simulink model "Simulate"  (R2024b)
settings: Solver=VariableStepAuto  StartTime=0.0  StopTime=Tf  FixedStep=Ti  MaxStep=Ti  RelTol=1e-6
undefined symbols (not defined in the file): CCMPC, CEMPC, DiscIntNeverNeededParam, dspblkCoreblockFVToolHelper, FOC, gcbh, IM, KF, LPF, M2C, plecs, PLL, RFT, TEB, Ti, Ts
libraries: slpidlib x4, spsdq0toAlphaBetaZeroLib x3, dspstat3 x2, spsAlphaBetaZerotoabcLib x2, embmathops x1, spsabctodq0Lib x1, spsAlphaBetaZerotodq0Lib x1, spsabctoAlphaBetaZeroLib x1
(part 2 of 2)

== matlab function Simulate/Energy balance1 ==
  data: Ec input; Vc input; VB input; IB input; ie_ref output; vo_ref output; flag output; J output; Nac output; Tex output; M2C parameter; CEMPC parameter
function [ie_ref, vo_ref, flag, J, Nac, Tex] = EMPC(Ec, Vc, VB, IB, M2C, CEMPC)
%#codegen

persistent Ts m n Np K MI NN NN1 NN2 ONE Nl is_max Vc_m_ref2 Ec_m_ref2 Hu_z1 Aineq_z1 Hu_z2 Aineq_z2 Hu_o Aineq_o lambda_z lambda_o iA_z1 iA_z2 iA_o options_z options_o
if isempty(Ts)
    Ts        = CEMPC.Ts;
    m         = M2C.m;
    n         = M2C.n;
    Np        = CEMPC.Np;
    K         = CEMPC.K;
    MI        = CEMPC.MI;
    NN        = CEMPC.NN;
    NN1       = CEMPC.NN1;
    NN2       = CEMPC.NN2;
    ONE       = CEMPC.ONE;
    Nl        = CEMPC.Nl;
    is_max    = M2C.is_max;
    Vc_m_ref2 = M2C.Vc_m_ref^2;
    Ec_m_ref2 = M2C.Ec_m_ref^2;
    Hu_z1     = CEMPC.Hu_z1;
    Aineq_z1  = CEMPC.Aineq_z1;
    Hu_z2     = CEMPC.Hu_z2;
    Aineq_z2  = CEMPC.Aineq_z2;
    Hu_o      = CEMPC.Hu_o;
    Aineq_o   = CEMPC.Aineq_o;
    lambda_z  = CEMPC.lambda_z;
    lambda_o  = CEMPC.lambda_o;
    iA_z1     = false(size(zeros(2 * m * Np, 1)));
    iA_z2     = false(size(zeros(2 * m * Np, 1)));
    iA_o      = false(size(zeros(2 * Np, 1)));
    options_z                     = mpcActiveSetOptions;
    options_z.MaxIterations       = 20;
    options_z.ConstraintTolerance = 1e-4;
    options_o                     = mpcActiveSetOptions;
    options_o.MaxIterations       = 10;
    options_o.ConstraintTolerance = 1e-4;
end

tic

% Preallocation
vo_ref_temp = zeros(Np, 1);
ie_ref_temp = zeros(n*Np, 1);
ie1_ref_temp = zeros(Np, 1);
ie2_ref_temp = zeros(Np, 1);
iz1_ref_temp = zeros(m*Np, 1);
iz2_ref_temp = zeros(m*Np, 1);
flag_z1 = int32(0);
flag_z2 = int32(0);
flag_o = int32(0);
vs_temp = zeros(m*Np, 1);
is_temp = zeros(m*Np, 1);

for l = 1:Nl
    %%%% LICCs subproblems J_z1 = Jx_z1 + Ju_z1, J_z2 = Jx_z2 + Ju_z2

    % Initialization
    vs_temp(:) = VB(:) + ONE * vo_ref_temp; % Cluster voltages

    %%% 1st LICC
    % Initialization
    iz2_ref_temp = NN2 * ie2_ref_temp; % 2nd circulating current

    % Linear model matrices
    E = Ts * K * diag(vs_temp); % Disturbances matrix
    B = E * NN1;                % Input matrix
    P = IB(:) + iz2_ref_temp;   % Disturbances

    % State reference tracking Jx_z1, quadratic and linear terms
    Hx_z1 = 2 * B' * MI * B / Ec_m_ref2;
    fx_z1 = 2 * B' * MI * (repmat(Ec, Np, 1) + E * P) / Ec_m_ref2;

    % Control action penalization Ju_z1, linear term
    fu_z1 = 2 * NN1' * P / is_max^2;

    % Total cost function J_z
    H_z1 = Hx_z1 + lambda_z * Hu_z1;
    f_z1 = fx_z1 + lambda_z * fu_z1;
    H_z1 = (H_z1 + H_z1') / 2;

    % Constraints
    ub      =  is_max - P;
    lb      = -is_max - P;
    bineq_z1 = [ub; -lb];

    % Solve
    [ie1_ref_temp, flag_z1, iA_z1] = mpcActiveSetSolver(H_z1, f_z1, Aineq_z1, bineq_z1, zeros(0, Np), zeros(0, 1), iA_z1, options_z);

    %%% 2nd LICC
    % Initialization
    iz1_ref_temp = NN1 * ie1_ref_temp; % 1nd circulating current

    % Linear model matrices
    E = Ts * K * diag(vs_temp); % Disturbances matrix
    B = E * NN2;                % Input matrix
    P = IB(:) + iz1_ref_temp;   % Disturbances

    % State reference tracking Jx_z2, quadratic and linear terms
    Hx_z2 = 2 * B' * MI * B / Ec_m_ref2;
    fx_z2 = 2 * B' * MI * (repmat(Ec, Np, 1) + E * P) / Ec_m_ref2;

    % Control action penalization Ju_z2, linear term
    fu_z2 = 2 * NN2' * P / is_max^2;

    % Total cost function J_z
    H_z2 = Hx_z2 + lambda_z * Hu_z2;
    f_z2 = fx_z2 + lambda_z * fu_z2;
    H_z2 = (H_z2 + H_z2') / 2;

    % Constraints
    ub       =  is_max - P;
    lb       = -is_max - P;
    bineq_z2 = [ub; -lb];

    % Solve
    [ie2_ref_temp, flag_z2, iA_z2] = mpcActiveSetSolver(H_z2, f_z2, Aineq_z2, bineq_z2, zeros(0, Np), zeros(0, 1), iA_z2, options_z);

    %%%% CMV subproblem Jo = Jx_o + Ju_o

    % Initialization
    iz1_ref_temp = NN1 * ie1_ref_temp;
    iz2_ref_temp = NN2 * ie2_ref_temp;
    iz_ref_temp = iz1_ref_temp + iz2_ref_temp;
    is_temp = IB(:) + iz_ref_temp;

    % Linear model matrices
    E = Ts * K * diag(is_temp); % Distrubances matrix
    B = E * ONE;                % Input matrix
    P = VB(:);                  % Distrubances

    % State reference tracking Jx_o, quadratic and linear terms 
    Hx_o = 2 * B' * MI * B / Ec_m_ref2;
    fx_o = 2 * B' * MI * (repmat(Ec, Np, 1) + E * P) / Ec_m_ref2;

    % Control action penalization Jo_u
    fu_o = zeros(Np, 1) / Vc_m_ref2;

    % Total cost function J_o
    H_o = Hx_o + lambda_o * Hu_o;
    f_o = fx_o + lambda_o * fu_o;
    H_o = (H_o + H_o') / 2;

    % Constraints
    ub = min([Vc(1:3); 0; 0; 0] - VB, [], 1)';
    lb = max([0; 0; 0; -Vc(4:6)] - VB, [], 1)';
    bineq_o = [ub; -lb];

    % Solve
    [vo_ref_temp, flag_o, iA_o] = mpcActiveSetSolver(H_o, f_o, Aineq_o, bineq_o, zeros(0, Np), zeros(0, 1), iA_o, options_o);
end

% ie_ref = ie_ref_temp(1:n);
ie_ref = ie_ref_temp(1:2);
vo_ref = vo_ref_temp(1);

vs_temp = VB(:) + ONE * vo_ref_temp;
Ec_pred = Ec + Ts * reshape(vs_temp .* is_temp, m, Np);
Ec_pred = Ec_pred(:);
J_E = sum((Ec_pred - mean(Ec_pred)).^2) / Ec_m_ref2;
J_i = sum(is_temp.^2) / is_max^2;
J_v = sum(vo_ref_temp.^2) / Vc_m_ref2;
J_T = J_E + lambda_z * J_i + lambda_o * J_v;

flag = [flag_z1, flag_z2, flag_o];
J = [J_E, J_i, J_v, J_T];
Nac = [sum(iA_z1), sum(iA_z2), sum(iA_o)];

Tex = toc;
end

% Hx = 2 * B' * B / M2C.Ec_m_ref^2;
% fx = 2 * B' * (repmat(x-mean(x), CEMPC.Np, 1) + E * P) / M2C.Ec_m_ref^2;

== matlab function Simulate/M2C+IM Average Model ==
  data: vs input; vB input; Fr_ab input; wm input; iu output; M2C parameter; CCMPC parameter; im output; ie output; Vc output; RFT parameter
function [iu, im, ie, Vc] = DM2C(vs, vB, Fr_ab, wm, M2C, CCMPC, RFT)

% DM2C: Decoupled M2C

persistent Ec m nx x Ad Bd integrated Tab2abc pinvA N Vdc Ts C
if isempty(Ec)
    m = M2C.m;
    Ec = M2C.Ec_m_ref * ones(m, 1);
    nx = CCMPC.nx;
    x = zeros(nx, 1);
    Ad = CCMPC.Ad;
    Bd = CCMPC.Bd;
    integrated = CCMPC.integrated;
    Tab2abc = RFT.ab2abc;
    pinvA = M2C.pinvA;
    N = M2C.N;
    Vdc = M2C.Vdc;
    Ts = CCMPC.Ts;
    C = M2C.C;
end

Es = CCMPC.Es;
Es(2, 3) = Es(2, 3)*wm;
Es(3, 2) = Es(3, 2)*wm;
Ed = integrated*Es;

p = [Vdc;
     Fr_ab;
     vB];

x = Ad * x + Bd * vs + Ed * p;

iu = x(1);
im = Tab2abc * x(2:3);
ie = x(2:3);

ixy = [iu;
      -iu;
      -im];
iB = pinvA * ixy;
iz = N * ie;
is = iB + iz;

Ec = Ec + Ts * vs .* is;

Vc = zeros(6, 1);
Vc(:) = sqrt(2 / C * Ec);

== matlab function Simulate/Energy balance ==
  data: Ec input; Vc input; VB input; IB input; ie_ref output; vo_ref output; flag output; J output; Nac output; Tex output; M2C parameter; CEMPC parameter
function [ie_ref, vo_ref, flag, J, Nac, Tex] = EMPC(Ec, Vc, VB, IB, M2C, CEMPC)
%#codegen

persistent Ts m n Np K MI NN ONE Nl is_max Vc_m_ref2 Ec_m_ref2 Hu_z Aineq_z lambda_z Hu_o Aineq_o lambda_o iA_z iA_o options_z options_o
if isempty(iA_z)
    Ts        = CEMPC.Ts;
    m         = M2C.m;
    n         = M2C.n;
    Np        = CEMPC.Np;
    K         = CEMPC.K;
    MI        = CEMPC.MI;
    NN        = CEMPC.NN;
    ONE       = CEMPC.ONE;
    Nl        = CEMPC.Nl;
    is_max    = M2C.is_max;
    Vc_m_ref2 = M2C.Vc_m_ref^2;
    Ec_m_ref2 = M2C.Ec_m_ref^2;
    Hu_z      = CEMPC.Hu_z;
    Aineq_z   = CEMPC.Aineq_z;
    lambda_z  = CEMPC.lambda_z;
    Hu_o      = CEMPC.Hu_o;
    Aineq_o   = CEMPC.Aineq_o;
    lambda_o  = CEMPC.lambda_o;
    iA_z      = false(size(zeros(2 * m * Np, 1)));
    iA_o      = false(size(zeros(2 * Np, 1)));
    options_z                     = mpcActiveSetOptions;
    options_z.MaxIterations       = 20;
    options_z.ConstraintTolerance = 1e-4;
    options_o                     = mpcActiveSetOptions;
    options_o.MaxIterations       = 10;
    options_o.ConstraintTolerance = 1e-4;
end

tic

% Preallocation
vo_ref_temp = zeros(Np, 1);
ie_ref_temp = zeros(n*Np, 1);
flag_z = int32(0);
flag_o = int32(0);
vs_temp = zeros(m*Np, 1);
is_temp = zeros(m*Np, 1);

for l = 1:Nl
    %%% LICCs subproblem Jz = Jz_x + Jz_u

    % Initialization
    % vs_temp(:) = VB(:) + ONE * vo_ref_temp;
    vs_temp = VB + vo_ref_temp';
    vs_temp = vs_temp(:);

    % Linear model matrices
    E = Ts * K * diag(vs_temp); % Disturbances matrix
    B = E * NN;                 % Input matrix
    P = IB(:);                  % Disturbances

    % State reference tracking Jx_z, quadratic and linear terms 
    Hx_z = 2 * B' * MI * B / Ec_m_ref2;
    fx_z = 2 * B' * MI * (repmat(Ec, Np, 1) + E * P) / Ec_m_ref2;

    % Control action penalization Ju_z, linear term
    fu_z = 2 * NN' * IB(:) / is_max^2;

    % Total cost function J_z
    H_z = Hx_z + lambda_z * Hu_z;
    f_z = fx_z + lambda_z * fu_z;
    H_z = (H_z + H_z') / 2;

    % Constraints
    ub      =  is_max - IB(:);
    lb      = -is_max - IB(:);
    bineq_z = [ub; -lb];

    % Solve
    [ie_ref_temp, flag_z, iA_z] = mpcActiveSetSolver(H_z, f_z, Aineq_z, bineq_z, zeros(0, n*Np), zeros(0, 1), iA_z, options_z);

    %%% CMV subproblem Jo = Jo_x + Jo_u

    % Initialization
    is_temp = IB(:) + NN * ie_ref_temp;

    % Linear model matrices
    E = Ts * K * diag(is_temp); % Distrubances matrix
    B = E * ONE;                % Input matrix
    P = VB(:);                  % Distrubances

    % State reference tracking Jx_o, quadratic and linear terms 
    Hx_o = 2 * B' * MI * B / Ec_m_ref2;
    fx_o = 2 * B' * MI * (repmat(Ec, Np, 1) + E * P) / Ec_m_ref2;

    % Control action penalization Jo_u
    fu_o = zeros(Np, 1) / Vc_m_ref2;

    % Total cost function J_o
    H_o = Hx_o + lambda_o * Hu_o;
    f_o = fx_o + lambda_o * fu_o;
    H_o = (H_o + H_o') / 2;

    % Constraints
    ub = min([Vc(1:3); 0; 0; 0] - VB, [], 1)';
    lb = max([0; 0; 0; -Vc(4:6)] - VB, [], 1)';
    bineq_o = [ub; -lb];

    % Solve
    [vo_ref_temp, flag_o, iA_o] = mpcActiveSetSolver(H_o, f_o, Aineq_o, bineq_o, zeros(0, Np), zeros(0, 1), iA_o, options_o);
end

% ie_ref = ie_ref_temp(1:n);
ie_ref = ie_ref_temp(1:2);
vo_ref = vo_ref_temp(1);

if and(0 < flag_z, 0 < flag_o)
    flag_T = 1;
else
    flag_T = -3;
end

vs_temp = VB(:) + ONE * vo_ref_temp;
Ec_pred = Ec + Ts * reshape(vs_temp .* is_temp, m, Np);
Ec_pred = Ec_pred(:);
J_E = sum((Ec_pred - mean(Ec_pred)).^2) / Ec_m_ref2;
J_i = sum(is_temp.^2) / is_max^2;
J_v = sum(vo_ref_temp.^2) / Vc_m_ref2;
J_T = J_E + lambda_z * J_i + lambda_o * J_v;

flag = [flag_z, flag_o, flag_T];
J = [J_E, J_i, J_v, J_T];
Nac = [sum(iA_z), sum(iA_o)];

Tex = toc;
end

== matlab function Simulate/Subsystem/MATLAB Function ==
  data: Vc input; vo_max output; vB input; vo_min output
function [vo_max, vo_min] = vo_lim(Vc, vB)

vo_max = min([Vc(1:3); zeros(3, 1)] - vB);
vo_min = max([zeros(3, 1); -Vc(4:6)] - vB);

== matlab function Simulate/Current control Converter only ==
  data: is_ref input; vo_ref input; vs_ref input; is input; vs output; Vc input; vB input; flag output; J output; Nac output; Tex output; M2C parameter; CCMPC parameter
function [vs, flag, J, Nac, Tex] = CMPC(is_ref, vo_ref, vs_ref, is, Vc, vB, M2C, CCMPC)
%#codegen

% CMPC: Cluster Current Model Predictive Control

% vs:   control action
% flag: solver verbose
% J:    cost function
% Nac:  # of active constraints
% Tex:  Execution time

% Initialization

persistent Ad Bd is_max Vc_m_ref lambda m Hx Hu H Aineq iA options
if isempty(Ad)
    Ad       = CCMPC.Ad;                  % Discrete state matrix
    Bd       = CCMPC.Bd;                  % Discrete input matrix
    is_max   = M2C.is_max;                % Max. cluster current
    Vc_m_ref = M2C.Vc_m_ref;              % Max. cluster capacitor voltage
    lambda   = CCMPC.lambda;              % Control effort weighting factor
    m        = M2C.m;                     % # of converter clusters
    Hx       = CCMPC.Hx;                  % Reference tracking hessian
    Hu       = CCMPC.Hu;                  % Control effort hessian
    H        = CCMPC.H;                   % Total hessian
    Aineq    = CCMPC.Aineq;               % Control actions constraints matrix
    iA       = false(size(Aineq, 1), 1);  % Active constraints
    options  = mpcActiveSetOptions;       % mpcActiveSetSolver options
    options.MaxIterations       = 100;
    options.ConstraintTolerance = 1.0e-5;
end

tic

% Reference tracking linear term, normalized
fx = 2 * Bd' * (-is_ref + Ad * is - Bd * vB) / is_max^2;

% Control effort linear term, normalized
fu = -2 * vs_ref / Vc_m_ref^2;

% Total weighted linear term
f = fx + lambda * fu;

% Control action constraints
ub    = [Vc(1:3); 0; 0; 0] + vo_ref;
lb    = [0; 0; 0; -Vc(4:6)] + vo_ref;
bineq = [ub; -lb];

% Solve
[vsp, flag, iA, ~] = mpcActiveSetSolver(H, f, Aineq, bineq, zeros(0, m), zeros(0, 1), iA, options);
vs = vsp - vo_ref;

% Control summary
Tex = toc;
Nac = sum(iA);
Jx = vsp' * Hx * vsp + fx' * vsp;
Ju = vsp' * Hu * vsp + fu' * vsp;
J  =  Jx + lambda * Ju;
end

== matlab function Simulate/Predict basic current and voltages ==
  data: VB output; vxy input; ixy input; wy input; RFT parameter; M2C parameter; CEMPC parameter; IB output
function [VB, IB] = pred(vxy, ixy, wy, RFT, M2C, CEMPC)
%#codegen

% vxy: (p+q) x Np
% ixy: (p+q) x Np
% VB: m x Np
% IB: m x Np

persistent p m Np Ts Tab2abc Tabc2ab A pinvA
if isempty(p)
    p       = M2C.p;
    m       = M2C.m;
    Np      = CEMPC.Np;
    Ts      = CEMPC.Ts;
    Tab2abc = RFT.ab2abc;
    Tabc2ab = RFT.abc2ab;
    A       = M2C.A;
    pinvA   = M2C.pinvA;
end

if Np > 1

    %%% Input port
    VX = repmat(vxy(1:p), 1, Np-1);
    IX = repmat(ixy(1:p), 1, Np-1);

    %%% Output port
    % Rotation matrix
    angles   = (1:Np-1) * (wy * Ts);
    cos_vals = cos(angles);
    sin_vals = sin(angles);
    ROTy     = reshape([cos_vals; -sin_vals; sin_vals; cos_vals], 2, 2*(Np-1))';

    % Predict
    VY = Tab2abc * reshape(ROTy * Tabc2ab * vxy(p+1:end), 2, Np-1);
    IY = Tab2abc * reshape(ROTy * Tabc2ab * ixy(p+1:end), 2, Np-1);

    %%% Predictions formatting
    
    % Concatenate input/output predictions
    VXY = [VX; VY];
    IXY = [IX; IY];
    
    % Add actual measurement as first predicted step
    VXY = [vxy, VXY];
    IXY = [ixy, IXY];
else
    VXY = vxy;
    IXY = ixy;
end

% VB = zeros(m, Np);
% IB = zeros(m, Np);
VB = zeros(6, 30);
IB = zeros(6, 30);

VB(:) = A' * VXY;
IB(:) = pinvA * IXY;
end

== matlab function Simulate/Steady state cluster voltage reference ==
  data: vs_ref output; im_ref input; iB_ref input; vB input; wy input; RFT parameter; M2C parameter
function vs_ref = get_vs_ref(im_ref, iB_ref, vB, wy, RFT, M2C)
%#codegen

% Steady state cluster voltage reference

persistent rot Tabc2ab Tab2abc pinvA invBs As
if isempty(rot)
    rot = RFT.rot;
    Tabc2ab = RFT.abc2ab;
    Tab2abc = RFT.ab2abc;
    pinvA = M2C.pinvA;
    invBs = M2C.invBs;
    As = M2C.As;
end

iy_ref = -im_ref;
dix_ref   = [0; 0];
iyab_ref  = Tabc2ab * iy_ref;
diyab_ref = wy * rot * iyab_ref;
diy_ref   = Tab2abc * diyab_ref;
dixy_ref  = [dix_ref; diy_ref];
diB_ref   = pinvA * dixy_ref;
vs_ref    = vB + invBs * (diB_ref - As * iB_ref);
end

== matlab function Simulate/MATLAB Function ==
  data: F output; t input; w output; IM parameter
function [F, w]= IM_ref(t, IM)

% IM_ref: Induction machine flux and speed references

% F: d-axis rotor flux
% w: mechanical speed

persistent wN wi wf ti_w tf_w dw FN Fi Ff ti_F tf_F dF
if isempty(wN)
    wN   = IM.wN;
    ti_w = 2;
    tf_w = 3;
    wi   = 0;
    wf   = wN/2;
    dw   = (wf - wi) / (tf_w - ti_w);

    FN = IM.FrN;
    ti_F = 0;
    tf_F = 1.5;
    Fi = 0;
    Ff = FN;
    dF = (Ff - Fi) / (tf_F - ti_F);
end

if t < ti_w
    w = wi;
elseif t < tf_w
    w = (t - ti_w) * dw;
else
    w = wf;
end

if t < ti_F
    F = Fi;
elseif t < tf_F
    F = (t - ti_F) * dF;
else
    F = Ff;
end

end

== matlab function Simulate/Kalman Filter ==
  data: im output; Fr output; wm output; Te output; yt input; ut input; KF parameter; Tex output; IM parameter; NIS output
function [im, Fr, wm, Te, Tex, NIS] = EKF(yt, ut, KF, IM)
%#codegen

persistent xt_est_apriori SIGt_apriori Q R Bd C kT np Inx
if isempty(xt_est_apriori)
    xt_est_apriori = KF.x1_mu;
    SIGt_apriori   = KF.SIG1;
    Q  = KF.Q;
    R  = KF.R;
    Bd = KF.Bd;
    C  = KF.C;
    kT = IM.kT;
    np = IM.np;
    Inx = eye(KF.nx);
end

tic

% xt_est = zeros(nx, 1);
xt_est = zeros(5, 1);

%% Measurement update
Kt = SIGt_apriori * C' / (R + C * SIGt_apriori * C');
yt_est = C * xt_est_apriori;
xt_est(:) = xt_est_apriori + Kt * (yt - yt_est);
SIGt = (Inx - Kt * C) * SIGt_apriori;

%% NIS (Normalized Innovation Squared)
v   = yt - yt_est;
S   = R + C * SIGt_apriori * C';
Lns = chol(S, 'lower');
t   = Lns'\v;
NIS = t' * t;

%% System matrices actualization
ima  = xt_est(1);
imb  = xt_est(2);
Fra  = xt_est(3);
Frb  = xt_est(4);
we   = xt_est(5);

% State matrix
Ad = KF.Ad;
Ad(1, 4) = Ad(1, 4) * we;
Ad(2, 3) = Ad(2, 3) * we;
Ad(3, 4) = Ad(3, 4) * we;
Ad(4, 3) = Ad(4, 3) * we;
Ad(5, 1) = Ad(5, 1) * Frb;
Ad(5, 2) = Ad(5, 2) * Fra;

% Jacobian
Adt = KF.Adt;
Adt(1, 4) = Ad(1, 4);
Adt(2, 3) = Ad(2, 3);
Adt(3, 4) = Ad(3, 4);
Adt(4, 3) = Ad(4, 3);
Adt(5, 1) = Ad(5, 1);
Adt(5, 2) = Ad(5, 2);
Adt(1, 5) = Adt(1, 5) * Frb;
Adt(2, 5) = Adt(2, 5) * Fra;
Adt(3, 5) = Adt(3, 5) * Frb;
Adt(4, 5) = Adt(4, 5) * Fra;
Adt(5, 3) = Adt(5, 3) * imb;
Adt(5, 4) = Adt(5, 4) * ima;

%% Temporal update
xt1_est = Ad * xt_est + Bd * ut;
% yt1_est = C * xt1_est;
SIGt1 = Q + Adt * SIGt * Adt';
SIGt_apriori = SIGt1;
xt_est_apriori = xt1_est;

%% Output
im = xt1_est(1:2);
Fr = xt1_est(3:4);
wm = xt1_est(5) / np;
Te = -kT * (Fr(2) * im(1) - Fr(1) * im(2));
Tex = toc;
